simulink library "biogas"  (Simulink 7.8)
settings: Solver=ode45  StartTime=0.0  StopTime=10.0  RelTol=1e-3
undefined symbols (not defined in the file or in its folder): adm1_loadfcn, appendDATA, biogas, Callback_ADM1_gui, configdivider, configmixer, datasourcetypes, DEBUG, deltatime, gas2bhkwsplittypes, hydraulic_delay_loadfcn, init_biogas_plant_mdl, initstatetypes, kalman_loadfcn, lda_state_estimator_loadfcn, plant, plant_network, pump_energy_loadfcn, pump_stream_loadfcn, sensors, substrate, substrate_mixer_digester_loadfcn, substrate_network, volumeflowtypes
libraries: biogas x8, simulink x5
(part 2 of 2)

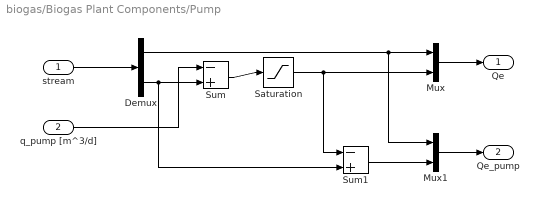
== system biogas/Biogas Plant Components/Pump ==
  stream : Inport
  q_pump [m^3/d] : Inport  Port=2
  Demux : Demux  Outputs=[33,1]
  Mux : Mux  Inputs=[33,1]
  Mux1 : Mux  Inputs=[33,1]
  Saturation : Saturate  UpperLimit=inf  LowerLimit=0
  Sum : Sum  Inputs=-+
  Sum1 : Sum  Inputs=-+
  Qe : Outport
  Qe_pump : Outport  Port=2
  wires:
  stream/1 -> Demux/1
  Mux/1 -> Qe/1
  Demux/1 -> Mux/1, Mux1/1
  q_pump [m^3/d]/1 -> Sum/1
  Demux/2 -> Sum/2, Sum1/2
  Sum/1 -> Saturation/1
  Saturation/1 -> Mux/2, Sum1/1
  Mux1/1 -> Qe_pump/1
  Sum1/1 -> Mux1/2

== system biogas/Biogas Plant Components/Pump (Energy) ==
  liquid [m^3/d] : Inport
  pump : S-Function  FunctionName=pump  Parameters=plant, substrate, appendDATA, char(plant.getDigesterID(fermenter_name - 1)), h_friction  EnableBusSupport=off
      mask Help: eval('web( ''html/pump.html'', ''-helpbrowser'')')
  pump energy per day [kWh/d] : Outport
  wires:
  pump/1 -> pump energy per day [kWh/d]/1
  liquid [m^3/d]/1 -> pump/1

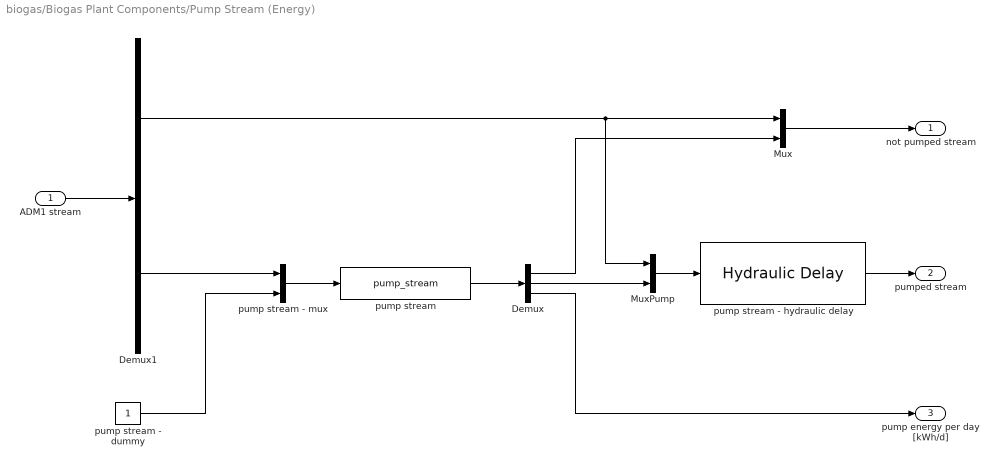
== system biogas/Biogas Plant Components/Pump Stream (Energy) ==
  ADM1 stream : Inport
  Demux : Demux  Outputs=3
  Demux1 : Demux  Outputs=[33,1]
  Mux : Mux  Inputs=[33,1]
  MuxPump : Mux  Inputs=[33,1]
  pump stream : S-Function  FunctionName=pump_stream  Parameters=plant, substrate, char(plant.getDigesterID(fermenter_name_start - 1)), char(plant.getDigesterID(fermenter_name_destiny - 1)), volumeflowtypes(volumeflow_type - 1), datasourcetypes(datasource_type - 1), sensors  EnableBusSupport=off
      mask Help: eval('web( ''html/pump.html'', ''-helpbrowser'')')
  pump stream - dummy : Constant
  pump stream - hydraulic delay : biogas/Biogas Plant Components/Hydraulic Delay  fermenter_name_start=--- Bitte Fermenter wählen ---  fermenter_name_destiny=--- Bitte Fermenter wählen ---  initstate_type=default  datasource_type=workspace  savestate=on  time_constant=1/24/30  V_min=100  isload=off  isbeingloaded=off  isbeingclosed=off  DEBUG_DISP=off
  pump stream - mux : Mux  Inputs=[1,1]
  not pumped stream : Outport
  pumped stream : Outport  Port=2
  pump energy per day [kWh/d] : Outport  Port=3
  wires:
  pump stream/1 -> Demux/1
  ADM1 stream/1 -> Demux1/1
  Demux1/1 -> Mux/1, MuxPump/1
  Demux/1 -> Mux/2
  Mux/1 -> not pumped stream/1
  Demux/2 -> MuxPump/2
  Demux/3 -> pump energy per day [kWh/d]/1
  pump stream - mux/1 -> pump stream/1
  Demux1/2 -> pump stream - mux/1
  pump stream - dummy/1 -> pump stream - mux/2
  MuxPump/1 -> pump stream - hydraulic delay/1
  pump stream - hydraulic delay/1 -> pumped stream/1

== system biogas/Biogas Plant Components/energy production ==
  biogas [m^3/d] : Inport
  Selector : Selector  InputPortWidth=plant.getNumCHPsD() + 1  IndexOptions=Index vector (dialog)  Indices=[1:plant.getNumCHPsD()]  OutputSizes=1
  Selector1 : Selector  InputPortWidth=plant.getNumCHPsD() + 1  IndexOptions=Index vector (dialog)  Indices=[plant.getNumCHPsD() + 1:plant.getNumCHPsD() + 1]  OutputSizes=1
  chps : S-Function  FunctionName=chps  Parameters=sensors, plant, gas2bhkwsplittypes(gas2bhkwsplit_type - 1)  EnableBusSupport=off
      mask Help: eval('web html/biogas_chp_plant.html')
  el. power [kW] : Outport
  excess gas [m^3/d] : Outport  Port=2
  wires:
  chps/1 -> Selector/1, Selector1/1
  biogas [m^3/d]/1 -> chps/1
  Selector/1 -> el. power [kW]/1
  Selector1/1 -> excess gas [m^3/d]/1

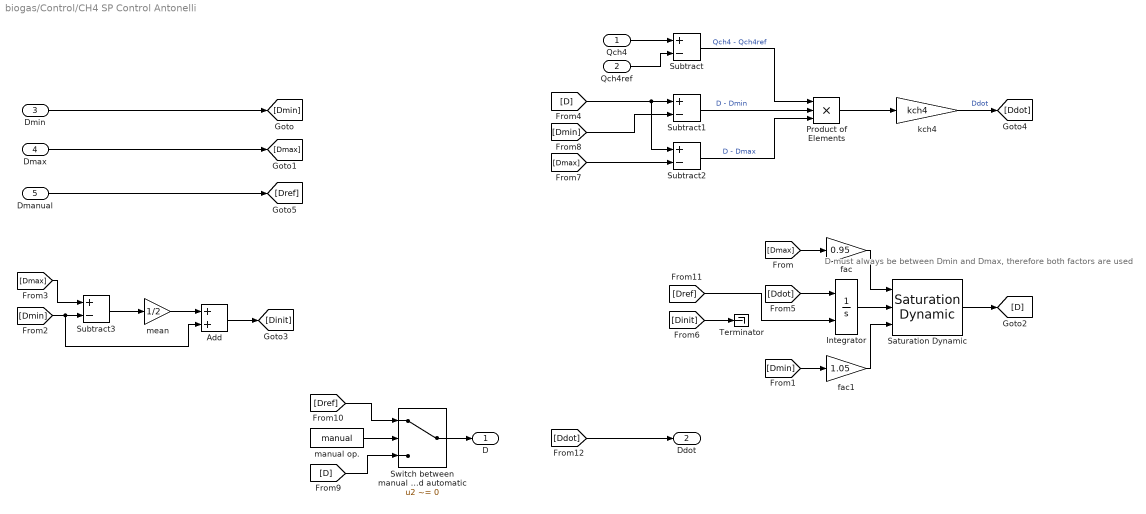
== system biogas/Control/CH4 SP Control Antonelli ==
  note: D must always be between Dmin and Dmax,
      | therefore both factors are used
  Qch4 : Inport
  Qch4ref : Inport  Port=2
  Dmin : Inport  Port=3
  Dmax : Inport  Port=4
  Dmanual : Inport  Port=5
  Add : Sum
  Integrator : Integrator  InitialConditionSource=external  InitialCondition=(0.1 - 0.0)/2
  Product of Elements : Product  Inputs=***
  Saturation Dynamic : simulink/Discontinuities/Saturation Dynamic  OutMin=[]  OutMax=[]  OutDataTypeStr=Inherit: Same as second input  OutDataType=fixdt(1, 16)  OutScaling=2^-10  DoSatur=off
  Subtract{,1..3} (4 alike) : Sum  Inputs=+-
  Switch between manual operation and automatic : Switch  Criteria=u2 ~= 0
  Terminator : Terminator
  fac : Gain  Gain=0.95
  fac1 : Gain  Gain=1.05
  kch4 : Gain  Gain=kch4
  manual op. : Constant  Value=manual
  mean : Gain  Gain=1/2
  D : Outport
  Ddot : Outport  Port=2
  wires:
  Dmax/1 -> [Dmax]
  Dmin/1 -> [Dmin]
  [Dref] -> Switch between manual operation and automatic/1
  [D] -> Switch between manual operation and automatic/3
  manual op./1 -> Switch between manual operation and automatic/2
  Switch between manual operation and automatic/1 -> D/1
  [Dmin] -> Subtract1/2
  [Dmax] -> Subtract2/2
  [Ddot] -> Integrator/1
  kch4/1 -> [Ddot]  "Ddot"
  Add/1 -> [Dinit]
  [D] -> Subtract2/1, Subtract1/1
  fac1/1 -> Saturation Dynamic/3
  fac/1 -> Saturation Dynamic/1
  [Dmax] -> Subtract3/1
  [Dmin] -> Add/2, Subtract3/2
  [Dmin] -> fac1/1
  [Dmax] -> fac/1
  mean/1 -> Add/1
  Dmanual/1 -> [Dref]
  Saturation Dynamic/1 -> [D]
  Subtract3/1 -> mean/1
  Qch4/1 -> Subtract/1
  Qch4ref/1 -> Subtract/2
  Subtract2/1 -> Product of Elements/3  "D - Dmax"
  Subtract1/1 -> Product of Elements/2  "D - Dmin"
  Subtract/1 -> Product of Elements/1  "Qch4 - Qch4ref"
  Product of Elements/1 -> kch4/1
  Integrator/1 -> Saturation Dynamic/2
  [Dref] -> Integrator/2
  [Ddot] -> Ddot/1
  [Dinit] -> Terminator/1

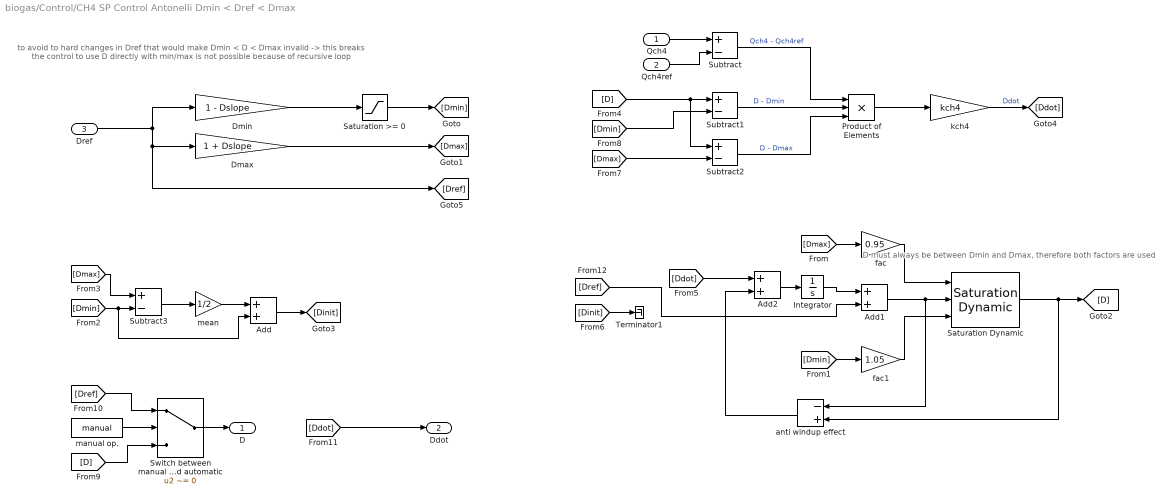
== system biogas/Control/CH4 SP Control Antonelli Dmin < Dref < Dmax ==
  note: D must always be between Dmin and Dmax,
      | therefore both factors are used
  note: to avoid to hard changes in Dref
      | that would make
      | Dmin < D < Dmax invalid
      | -> this breaks the control
      | to use D directly with min/max
      | is not possible because of recursive loop
  Qch4 : Inport
  Qch4ref : Inport  Port=2
  Dref : Inport  Port=3
  Add : Sum
  Add1 : Sum
  Add2 : Sum
  Dmax : Gain  Gain=1 + Dslope
  Dmin : Gain  Gain=1 - Dslope
  Integrator : Integrator
  Product of Elements : Product  Inputs=***
  Saturation Dynamic : simulink/Discontinuities/Saturation Dynamic  OutMin=[]  OutMax=[]  OutDataTypeStr=Inherit: Same as second input  OutDataType=fixdt(1, 16)  OutScaling=2^-10  DoSatur=off
  Saturation >= 0 : Saturate  UpperLimit=Inf  LowerLimit=0
  Subtract{,1..3} (4 alike) : Sum  Inputs=+-
  Switch between manual operation and automatic : Switch  Criteria=u2 ~= 0
  Terminator1 : Terminator
  anti windup effect : Sum  Inputs=-+
  fac : Gain  Gain=0.95
  fac1 : Gain  Gain=1.05
  kch4 : Gain  Gain=kch4
  manual op. : Constant  Value=manual
  mean : Gain  Gain=1/2
  D : Outport
  Ddot : Outport  Port=2
  wires:
  Product of Elements/1 -> kch4/1
  Subtract/1 -> Product of Elements/1  "Qch4 - Qch4ref"
  Subtract1/1 -> Product of Elements/2  "D - Dmin"
  Subtract2/1 -> Product of Elements/3  "D - Dmax"
  Qch4ref/1 -> Subtract/2
  Qch4/1 -> Subtract/1
  Subtract3/1 -> mean/1
  Saturation Dynamic/1 -> [D], anti windup effect/2
  Dref/1 -> Dmin/1, Dmax/1, [Dref]
  mean/1 -> Add/1
  [Dmax] -> fac/1
  [Dmin] -> fac1/1
  [Dmin] -> Subtract3/2, Add/2
  [Dmax] -> Subtract3/1
  fac/1 -> Saturation Dynamic/1
  fac1/1 -> Saturation Dynamic/3
  [D] -> Subtract1/1, Subtract2/1
  Add/1 -> [Dinit]
  kch4/1 -> [Ddot]  "Ddot"
  [Dmax] -> Subtract2/2
  [Dmin] -> Subtract1/2
  Switch between manual operation and automatic/1 -> D/1
  manual op./1 -> Switch between manual operation and automatic/2
  [D] -> Switch between manual operation and automatic/3
  [Dref] -> Switch between manual operation and automatic/1
  Dmin/1 -> Saturation >= 0/1
  Dmax/1 -> [Dmax]
  Saturation >= 0/1 -> [Dmin]
  [Ddot] -> Ddot/1
  [Dinit] -> Terminator1/1
  Integrator/1 -> Add1/1
  Add1/1 -> Saturation Dynamic/2, anti windup effect/1
  [Dref] -> Add1/2
  anti windup effect/1 -> Add2/2
  Add2/1 -> Integrator/1
  [Ddot] -> Add2/1

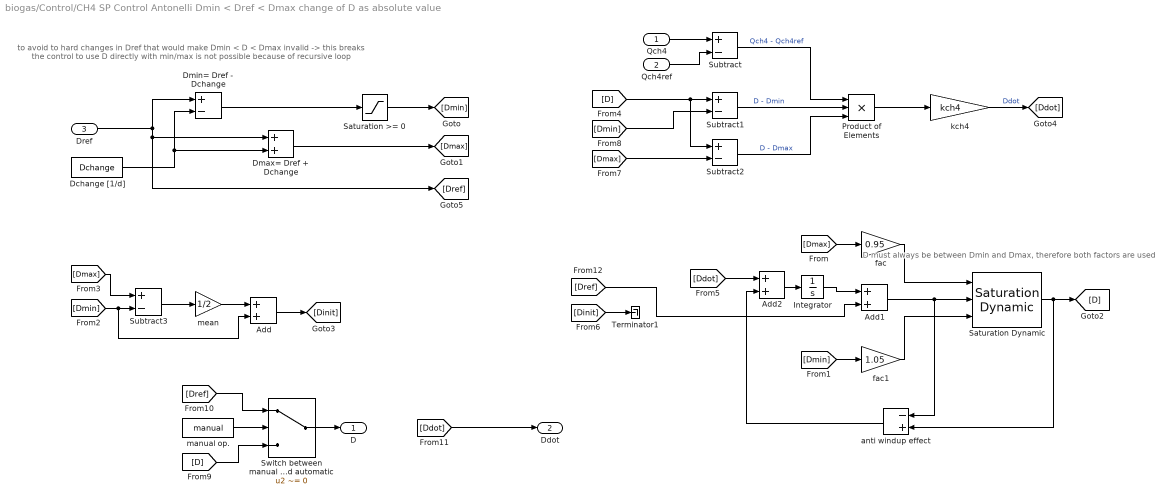
== system biogas/Control/CH4 SP Control Antonelli Dmin < Dref < Dmax change of D as absolute value ==
  note: to avoid to hard changes in Dref
      | that would make
      | Dmin < D < Dmax invalid
      | -> this breaks the control
      | to use D directly with min/max
      | is not possible because of recursive loop
  note: D must always be between Dmin and Dmax,
      | therefore both factors are used
  Qch4 : Inport
  Qch4ref : Inport  Port=2
  Dref : Inport  Port=3
  Add : Sum
  Add1 : Sum
  Add2 : Sum
  Dchange [1/d] : Constant  Value=Dchange
  Dmax= Dref + Dchange : Sum
  Dmin= Dref - Dchange : Sum  Inputs=+-
  Integrator : Integrator
  Product of Elements : Product  Inputs=***
  Saturation Dynamic : simulink/Discontinuities/Saturation Dynamic  OutMin=[]  OutMax=[]  OutDataTypeStr=Inherit: Same as second input  OutDataType=fixdt(1, 16)  OutScaling=2^-10  DoSatur=off
  Saturation >= 0 : Saturate  UpperLimit=Inf  LowerLimit=0
  Subtract{,1..3} (4 alike) : Sum  Inputs=+-
  Switch between manual operation and automatic : Switch  Criteria=u2 ~= 0
  Terminator1 : Terminator
  anti windup effect : Sum  Inputs=-+
  fac : Gain  Gain=0.95
  fac1 : Gain  Gain=1.05
  kch4 : Gain  Gain=kch4
  manual op. : Constant  Value=manual
  mean : Gain  Gain=1/2
  D : Outport
  Ddot : Outport  Port=2
  wires:
  [Dref] -> Add1/2
  Add1/1 -> Saturation Dynamic/2, anti windup effect/1
  Integrator/1 -> Add1/1
  [Dinit] -> Terminator1/1
  [Ddot] -> Ddot/1
  Saturation >= 0/1 -> [Dmin]
  Dmax= Dref + Dchange/1 -> [Dmax]
  Dmin= Dref - Dchange/1 -> Saturation >= 0/1
  [Dref] -> Switch between manual operation and automatic/1
  [D] -> Switch between manual operation and automatic/3
  manual op./1 -> Switch between manual operation and automatic/2
  Switch between manual operation and automatic/1 -> D/1
  [Dmin] -> Subtract1/2
  [Dmax] -> Subtract2/2
  kch4/1 -> [Ddot]  "Ddot"
  Add/1 -> [Dinit]
  [D] -> Subtract2/1, Subtract1/1
  fac1/1 -> Saturation Dynamic/3
  fac/1 -> Saturation Dynamic/1
  [Dmax] -> Subtract3/1
  [Dmin] -> Add/2, Subtract3/2
  [Dmin] -> fac1/1
  [Dmax] -> fac/1
  mean/1 -> Add/1
  Dref/1 -> [Dref], Dmax= Dref + Dchange/1, Dmin= Dref - Dchange/1
  Saturation Dynamic/1 -> [D], anti windup effect/2
  Subtract3/1 -> mean/1
  Qch4/1 -> Subtract/1
  Qch4ref/1 -> Subtract/2
  Subtract2/1 -> Product of Elements/3  "D - Dmax"
  Subtract1/1 -> Product of Elements/2  "D - Dmin"
  Subtract/1 -> Product of Elements/1  "Qch4 - Qch4ref"
  Product of Elements/1 -> kch4/1
  Dchange [1/d]/1 -> Dmin= Dref - Dchange/2, Dmax= Dref + Dchange/2
  Add2/1 -> Integrator/1
  [Ddot] -> Add2/1
  anti windup effect/1 -> Add2/2

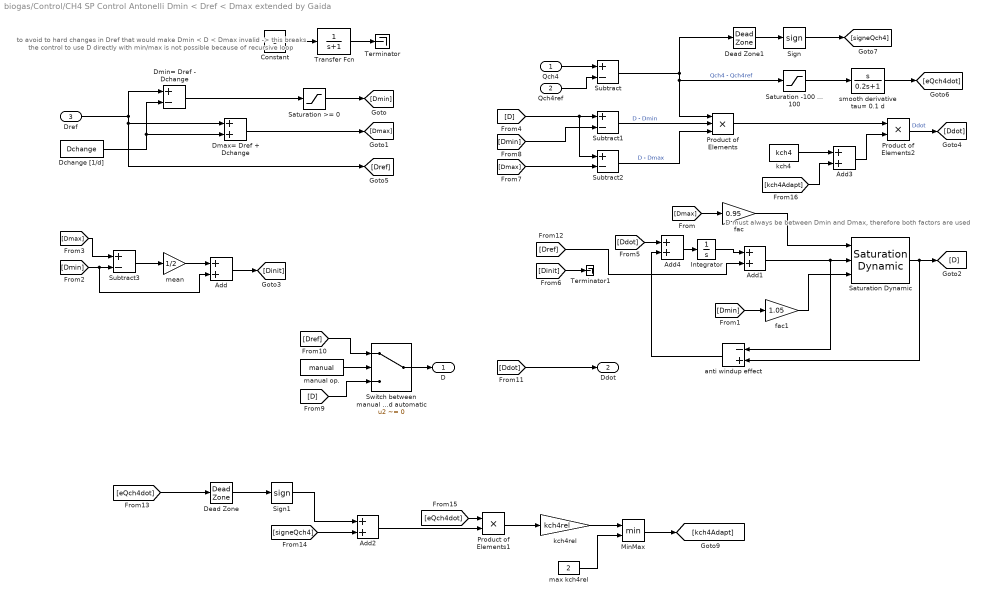
== system biogas/Control/CH4 SP Control Antonelli Dmin < Dref < Dmax extended by Gaida ==
  note: D must always be between Dmin and Dmax,
      | therefore both factors are used
  note: to avoid to hard changes in Dref
      | that would make
      | Dmin < D < Dmax invalid
      | -> this breaks the control
      | to use D directly with min/max
      | is not possible because of recursive loop
  Qch4 : Inport
  Qch4ref : Inport  Port=2
  Dref : Inport  Port=3
  Add{,1..4} (5 alike) : Sum
  Constant : Constant
  Dchange [1/d] : Constant  Value=Dchange
  Dead Zone : DeadZone  LowerValue=-0.001  UpperValue=0.001  SaturateOnIntegerOverflow=on
  Dead Zone1 : DeadZone  LowerValue=-0.001  UpperValue=0.001  SaturateOnIntegerOverflow=on
  Dmax= Dref + Dchange : Sum
  Dmin= Dref - Dchange : Sum  Inputs=+-
  Integrator : Integrator
  MinMax : MinMax  Inputs=2
  Product of Elements : Product  Inputs=***
  Product of Elements1 : Product  Inputs=**
  Product of Elements2 : Product  Inputs=**
  Saturation -100 ... 100 : Saturate  UpperLimit=100  LowerLimit=-100
  Saturation Dynamic : simulink/Discontinuities/Saturation Dynamic  OutMin=[]  OutMax=[]  OutDataTypeStr=Inherit: Same as second input  OutDataType=fixdt(1, 16)  OutScaling=2^-10  DoSatur=off
  Saturation >= 0 : Saturate  UpperLimit=Inf  LowerLimit=0
  Sign : Signum
  Sign1 : Signum
  Subtract{,1..3} (4 alike) : Sum  Inputs=+-
  Switch between manual operation and automatic : Switch  Criteria=u2 ~= 0
  Terminator : Terminator
  Terminator1 : Terminator
  Transfer Fcn : TransferFcn  Denominator=[1 1]
  anti windup effect : Sum  Inputs=-+
  fac : Gain  Gain=0.95
  fac1 : Gain  Gain=1.05
  kch4 : Constant  Value=kch4
  kch4rel : Gain  Gain=kch4rel
  manual op. : Constant  Value=manual
  max kch4rel : Constant  Value=2
  mean : Gain  Gain=1/2
  smooth derivative tau= 0.1 d : TransferFcn  Numerator=[1 0]  Denominator=[0.2 1]
  D : Outport
  Ddot : Outport  Port=2
  wires:
  Dchange [1/d]/1 -> Dmax= Dref + Dchange/2, Dmin= Dref - Dchange/2
  Product of Elements/1 -> Product of Elements2/1
  Subtract/1 -> Dead Zone1/1, Product of Elements/1, Saturation -100 ... 100/1  "Qch4 - Qch4ref"
  Subtract1/1 -> Product of Elements/2  "D - Dmin"
  Subtract2/1 -> Product of Elements/3  "D - Dmax"
  Qch4ref/1 -> Subtract/2
  Qch4/1 -> Subtract/1
  Subtract3/1 -> mean/1
  Saturation Dynamic/1 -> [D], anti windup effect/2
  Dref/1 -> Dmin= Dref - Dchange/1, Dmax= Dref + Dchange/1, [Dref]
  mean/1 -> Add/1
  [Dmax] -> fac/1
  [Dmin] -> fac1/1
  [Dmin] -> Subtract3/2, Add/2
  [Dmax] -> Subtract3/1
  fac/1 -> Saturation Dynamic/1
  fac1/1 -> Saturation Dynamic/3
  [D] -> Subtract1/1, Subtract2/1
  Add/1 -> [Dinit]
  Product of Elements2/1 -> [Ddot]  "Ddot"
  [Dmax] -> Subtract2/2
  [Dmin] -> Subtract1/2
  Switch between manual operation and automatic/1 -> D/1
  manual op./1 -> Switch between manual operation and automatic/2
  [D] -> Switch between manual operation and automatic/3
  [Dref] -> Switch between manual operation and automatic/1
  Dmin= Dref - Dchange/1 -> Saturation >= 0/1
  Dmax= Dref + Dchange/1 -> [Dmax]
  Constant/1 -> Transfer Fcn/1
  Transfer Fcn/1 -> Terminator/1
  Saturation >= 0/1 -> [Dmin]
  [Ddot] -> Ddot/1
  [Dinit] -> Terminator1/1
  Integrator/1 -> Add1/1
  Add1/1 -> Saturation Dynamic/2, anti windup effect/1
  [Dref] -> Add1/2
  smooth derivative tau= 0.1 d/1 -> [eQch4dot]
  Sign/1 -> [signeQch4]
  [eQch4dot] -> Dead Zone/1
  Sign1/1 -> Add2/1
  [signeQch4] -> Add2/2
  Add2/1 -> Product of Elements1/2
  [eQch4dot] -> Product of Elements1/1
  Product of Elements1/1 -> kch4rel/1
  kch4/1 -> Add3/1
  [kch4Adapt] -> Add3/2
  Add3/1 -> Product of Elements2/2
  Add4/1 -> Integrator/1
  [Ddot] -> Add4/1
  anti windup effect/1 -> Add4/2
  Dead Zone/1 -> Sign1/1
  Dead Zone1/1 -> Sign/1
  kch4rel/1 -> MinMax/1
  MinMax/1 -> [kch4Adapt]
  max kch4rel/1 -> MinMax/2
  Saturation -100 ... 100/1 -> smooth derivative tau= 0.1 d/1

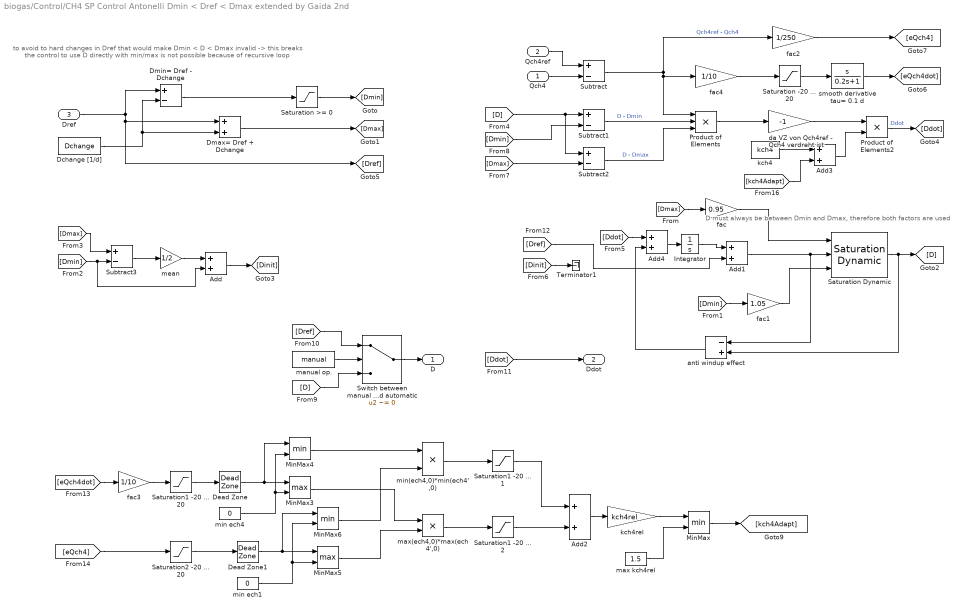
== system biogas/Control/CH4 SP Control Antonelli Dmin < Dref < Dmax extended by Gaida 2nd ==
  note: to avoid to hard changes in Dref
      | that would make
      | Dmin < D < Dmax invalid
      | -> this breaks the control
      | to use D directly with min/max
      | is not possible because of recursive loop
  note: D must always be between Dmin and Dmax,
      | therefore both factors are used
  Qch4 : Inport
  Qch4ref : Inport  Port=2
  Dref : Inport  Port=3
  Add{,1..4} (5 alike) : Sum
  Dchange [1/d] : Constant  Value=Dchange
  Dead Zone : DeadZone  LowerValue=-0.001  UpperValue=0.001  SaturateOnIntegerOverflow=on
  Dead Zone1 : DeadZone  LowerValue=-0.001  UpperValue=0.001  SaturateOnIntegerOverflow=on
  Dmax= Dref + Dchange : Sum
  Dmin= Dref - Dchange : Sum  Inputs=+-
  Integrator : Integrator
  MinMax : MinMax  Inputs=2
  MinMax3 : MinMax  Function=max  Inputs=2
  MinMax4 : MinMax  Inputs=2
  MinMax5 : MinMax  Function=max  Inputs=2
  MinMax6 : MinMax  Inputs=2
  Product of Elements : Product  Inputs=***
  Product of Elements2 : Product  Inputs=**
  Saturation -20 ... 20 : Saturate  UpperLimit=20  LowerLimit=-20
  Saturation Dynamic : simulink/Discontinuities/Saturation Dynamic  OutMin=[]  OutMax=[]  OutDataTypeStr=Inherit: Same as second input  OutDataType=fixdt(1, 16)  OutScaling=2^-10  DoSatur=off
  Saturation >= 0 : Saturate  UpperLimit=Inf  LowerLimit=0
  Saturation1 -20 ... 1 : Saturate  UpperLimit=20  LowerLimit=-20
  Saturation1 -20 ... 2 : Saturate  UpperLimit=20  LowerLimit=-20
  Saturation1 -20 ... 20 : Saturate  UpperLimit=20  LowerLimit=-20
  Saturation2 -20 ... 20 : Saturate  UpperLimit=20  LowerLimit=-20
  Subtract{,1..3} (4 alike) : Sum  Inputs=+-
  Switch between manual operation and automatic : Switch  Criteria=u2 ~= 0
  Terminator1 : Terminator
  anti windup effect : Sum  Inputs=-+
  da VZ von Qch4ref - Qch4 verdreht ist : Gain  Gain=-1
  fac : Gain  Gain=0.95
  fac1 : Gain  Gain=1.05
  fac2 : Gain  Gain=1/250
  fac3 : Gain  Gain=1/10
  fac4 : Gain  Gain=1/10
  kch4 : Constant  Value=kch4
  kch4rel : Gain  Gain=kch4rel
  manual op. : Constant  Value=manual
  max kch4rel : Constant  Value=1.5
  max(ech4,0)*max(ech4',0) : Product  Inputs=**
  mean : Gain  Gain=1/2
  min ech1 : Constant  Value=0
  min ech4 : Constant  Value=0
  min(ech4,0)*min(ech4',0) : Product  Inputs=**
  smooth derivative tau= 0.1 d : TransferFcn  Numerator=[1 0]  Denominator=[0.2 1]
  D : Outport
  Ddot : Outport  Port=2
  wires:
  Saturation -20 ... 20/1 -> smooth derivative tau= 0.1 d/1
  max kch4rel/1 -> MinMax/2
  MinMax/1 -> [kch4Adapt]
  kch4rel/1 -> MinMax/1
  anti windup effect/1 -> Add4/2
  [Ddot] -> Add4/1
  Add4/1 -> Integrator/1
  Add3/1 -> Product of Elements2/2
  [kch4Adapt] -> Add3/2
  kch4/1 -> Add3/1
  Add2/1 -> kch4rel/1
  [eQch4dot] -> fac3/1
  smooth derivative tau= 0.1 d/1 -> [eQch4dot]
  [Dref] -> Add1/2
  Add1/1 -> anti windup effect/1, Saturation Dynamic/2
  Integrator/1 -> Add1/1
  [Dinit] -> Terminator1/1
  [Ddot] -> Ddot/1
  Saturation >= 0/1 -> [Dmin]
  Dmax= Dref + Dchange/1 -> [Dmax]
  Dmin= Dref - Dchange/1 -> Saturation >= 0/1
  [Dref] -> Switch between manual operation and automatic/1
  [D] -> Switch between manual operation and automatic/3
  manual op./1 -> Switch between manual operation and automatic/2
  Switch between manual operation and automatic/1 -> D/1
  [Dmin] -> Subtract1/2
  [Dmax] -> Subtract2/2
  Product of Elements2/1 -> [Ddot]  "Ddot"
  Add/1 -> [Dinit]
  [D] -> Subtract2/1, Subtract1/1
  fac1/1 -> Saturation Dynamic/3
  fac/1 -> Saturation Dynamic/1
  [Dmax] -> Subtract3/1
  [Dmin] -> Add/2, Subtract3/2
  [Dmin] -> fac1/1
  [Dmax] -> fac/1
  mean/1 -> Add/1
  Dref/1 -> [Dref], Dmax= Dref + Dchange/1, Dmin= Dref - Dchange/1
  Saturation Dynamic/1 -> anti windup effect/2, [D]
  Subtract3/1 -> mean/1
  Subtract2/1 -> Product of Elements/3  "D - Dmax"
  Subtract1/1 -> Product of Elements/2  "D - Dmin"
  Subtract/1 -> fac2/1, Product of Elements/1, fac4/1  "Qch4ref - Qch4"
  Product of Elements/1 -> da VZ von Qch4ref - Qch4 verdreht ist/1
  Dchange [1/d]/1 -> Dmin= Dref - Dchange/2, Dmax= Dref + Dchange/2
  Qch4ref/1 -> Subtract/1
  Qch4/1 -> Subtract/2
  min ech4/1 -> MinMax3/2, MinMax4/2
  [eQch4] -> Saturation2 -20 ... 20/1
  min ech1/1 -> MinMax5/2, MinMax6/2
  MinMax4/1 -> min(ech4,0)*min(ech4',0)/1
  MinMax6/1 -> min(ech4,0)*min(ech4',0)/2
  min(ech4,0)*min(ech4',0)/1 -> Saturation1 -20 ... 1/1
  MinMax3/1 -> max(ech4,0)*max(ech4',0)/1
  MinMax5/1 -> max(ech4,0)*max(ech4',0)/2
  fac2/1 -> [eQch4]
  Dead Zone/1 -> MinMax3/1, MinMax4/1
  Dead Zone1/1 -> MinMax5/1, MinMax6/1
  max(ech4,0)*max(ech4',0)/1 -> Saturation1 -20 ... 2/1
  Saturation1 -20 ... 20/1 -> Dead Zone/1
  Saturation2 -20 ... 20/1 -> Dead Zone1/1
  fac3/1 -> Saturation1 -20 ... 20/1
  Saturation1 -20 ... 1/1 -> Add2/1
  Saturation1 -20 ... 2/1 -> Add2/2
  fac4/1 -> Saturation -20 ... 20/1
  da VZ von Qch4ref - Qch4 verdreht ist/1 -> Product of Elements2/1

== system biogas/Optimization/fitness sensor ==
  dummy : Constant  Value=0
  fitness sensor : S-Function  FunctionName=fitness_sensor  Parameters=sensors, plant, substrate, fitness_params  EnableBusSupport=off
  fitness : Outport
  wires:
  dummy/1 -> fitness sensor/1
  fitness sensor/1 -> fitness/1

== system biogas/Optimization/simulation killer ==
  max time : Inport
  kill_simulation : S-Function  FunctionName=kill_simulation  EnableBusSupport=off
  cur delta time : Outport
  wires:
  kill_simulation/1 -> cur delta time/1
  max time/1 -> kill_simulation/1

== system biogas/Prediction/Kalman Filter cont. ==
  Qin : Inport
  Kalman filter : S-Function  FunctionName=KalmanFilterContinuous  Parameters=DEBUG, deltatime, plant, plant.fermenter.ids(fermenter_name - 1), initstatetypes(initstate_type - 1), datasourcetypes(datasource_type - 1), @KalmanFilterCont_ADM1  EnableBusSupport=off
  x hat : Outport
  wires:
  Qin/1 -> Kalman filter/1
  Kalman filter/1 -> x hat/1

== system biogas/Prediction/LDA State Estimator ==
  LDA State Estimator block : S-Function  FunctionName=LDAStateEstimator  Parameters=plant, plant.fermenter.ids(fermenter_name - 1), 'Sac', DEBUG, deltatime  EnableBusSupport=off
  dummy : Constant  Value=0
  state estimate : Outport
  wires:
  LDA State Estimator block/1 -> state estimate/1
  dummy/1 -> LDA State Estimator block/1

== system biogas/Prediction/RF State Estimator ==
  RF State Estimator block : S-Function  FunctionName=RFStateEstimator  Parameters=plant, plant.fermenter.ids(fermenter_name - 1), 'Sac', DEBUG, deltatime  EnableBusSupport=off
  dummy : Constant  Value=0
  state estimate : Outport
  wires:
  dummy/1 -> RF State Estimator block/1
  RF State Estimator block/1 -> state estimate/1

== system biogas/Sensors/substrateflow sensor ==
  ADM1xp stream : Inport
  Selector : Selector  InputPortWidth=biogas.ADMstate.dim_stream  IndexOptions=Index vector (dialog)  Indices=[biogas.ADMstate.pos_Q]  OutputSizes=1
  substrate flow [m^3/d] : Outport
  wires:
  ADM1xp stream/1 -> Selector/1
  Selector/1 -> substrate flow [m^3/d]/1

== system biogas/Substrate Sources/Internal ==
  Create ADM stream Mix : Subsystem  mask{volumeflow_type='random', datasource_type='file'}
      mask prompts: volumeflow_type "volumeflow_type : type of the volume flow input data (e.g. 'random', 'const', 'user')"; datasource_type "source for the volumeflow data (datasource_type)"

== system biogas/Substrate Sources/Substrate Mixer (Digester) ==
  dilution rates : Inport
  Create ADM stream Mix : biogas/Substrate Sources/Internal/Create ADM stream Mix  volumeflow_type=volumeflowtypes(1,volumeflow_type - 1)  datasource_type=datasourcetypes(datasource_type - 1)
  Demux : Demux  Outputs=plant.getNumDigestersD()
  tag scope: main=global
  wires:
  Create ADM stream Mix/1 -> Demux/1
  Demux/1 -> [main]
  dilution rates/1 -> Create ADM stream Mix/1

== system biogas/Anaerobic Digestion Models/Internal/ADM1DE ==
  Qin : Inport
  ADM1 : S-Function  FunctionName=ADM1DE  Parameters=sensors, plant, substrate, substrate_network, plant_network, char(plant.getDigesterID(fermenter_name - 1)), initstatetypes(initstate_type - 1), datasourcetypes(datasource_type - 1), savestate  EnableBusSupport=off
  Select Gas : Selector  InputPortWidth=biogas.ADMstate.dim_stream + biogas.BioGas.n_gases  IndexOptions=Index vector (dialog)  Indices=[35:37]  OutputSizes=1
  Select Qe : Selector  InputPortWidth=biogas.ADMstate.dim_stream + biogas.BioGas.n_gases  IndexOptions=Index vector (dialog)  Indices=[1:biogas.ADMstate.dim_stream]  OutputSizes=1
  Gas : Outport
  Qe : Outport  Port=2
  wires:
  ADM1/1 -> Select Qe/1, Select Gas/1
  Qin/1 -> ADM1/1
  Select Qe/1 -> Qe/1
  Select Gas/1 -> Gas/1

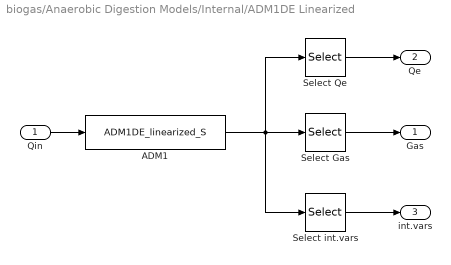
== system biogas/Anaerobic Digestion Models/Internal/ADM1DE Linearized ==
  Qin : Inport
  ADM1 : S-Function  FunctionName=ADM1DE_linearized_S  Parameters=DEBUG, deltatime, plant, plant.fermenter.ids(fermenter_name - 1), initstatetypes(initstate_type - 1), datasourcetypes(datasource_type - 1), savestate  EnableBusSupport=off
  Select Gas : Selector  InputPortWidth=34+3+64  IndexOptions=Index vector (dialog)  Indices=[35:37]  OutputSizes=1
  Select Qe : Selector  InputPortWidth=34+3+64  IndexOptions=Index vector (dialog)  Indices=[1:34]  OutputSizes=1
  Select int.vars : Selector  InputPortWidth=34+3+64  IndexOptions=Index vector (dialog)  Indices=[38:38+63]  OutputSizes=1
  Gas : Outport
  Qe : Outport  Port=2
  int.vars : Outport  Port=3
  wires:
  Select int.vars/1 -> int.vars/1
  Select Gas/1 -> Gas/1
  Select Qe/1 -> Qe/1
  Qin/1 -> ADM1/1
  ADM1/1 -> Select int.vars/1, Select Gas/1, Select Qe/1

== system biogas/Substrate Sources/Internal/Create ADM stream Mix ==
  In1 : Inport
  createADMstreamMix : S-Function  FunctionName=createADMstreamMix  Parameters=volumeflow_type, substrate_network, substrate, sensors, plant, datasource_type  EnableBusSupport=off
      mask Type: create daily hydrograph
      mask Help: eval('web( ''html/createdailyhydrograph_mat.html'', ''-helpbrowser'')')
  out : Outport
  wires:
  createADMstreamMix/1 -> out/1
  In1/1 -> createADMstreamMix/1
